simulink model "double_pendulum"  (R2021b)
settings: Solver=VariableStepAuto  StartTime=0.0  StopTime=10.0  RelTol=1e-3
values from neighbouring files (symbols this model uses):
  b1 = 7.7210    (= 7.721)    [benchmark_dbl_pend.m]    (also in dbl_pend_upup_stab_RL.m = 4.8)
  b2 = 2.337424773114795e-05    (= 2.33742477311e-05)    [benchmark_dbl_pend.m]    (also in dbl_pend_upup_stab_RL.m = 0.0002)
  bounds_th1 = [-pi, 3*pi]    [dbl_pend_upup_stab_RL.m]
  c1 = -0.0320    (= -0.032)    [benchmark_dbl_pend.m]    (also in dbl_pend_upup_stab_RL.m = -0.04)
  c2 = 0.053232610186913    (= 0.0532326101869)    [benchmark_dbl_pend.m]    (also in dbl_pend_upup_stab_RL.m = 0.06)
  I1 = 0.0888    [benchmark_dbl_pend.m]    (also in dbl_pend_upup_stab_RL.m = 0.074)
  I2 = 9.5326e-05    [benchmark_dbl_pend.m]    (also in dbl_pend_upup_stab_RL.m = 0.00012)
  km = 53.049364666321930    (= 53.0493646663)    [benchmark_dbl_pend.m]    (also in dbl_pend_upup_stab_RL.m = 50)
  l1 = 0.1    [benchmark_dbl_pend.m]    (also in dbl_pend_upup_stab_RL.m)
  l2 = 0.1    [benchmark_dbl_pend.m]    (also in dbl_pend_upup_stab_RL.m)
  m1 = 0.125    [benchmark_dbl_pend.m]    (also in dbl_pend_upup_stab_RL.m)
  m2 = 0.0493    [benchmark_dbl_pend.m]    (also in dbl_pend_upup_stab_RL.m = 0.05)
  tau_e = 0.014999999999983    (= 0.015)    [benchmark_dbl_pend.m]    (also in dbl_pend_upup_stab_RL.m = 0.03)
  w = [1, 1, 0.05, 0.1]    [dbl_pend_upup_stab_RL.m]
undefined symbols (not defined in the file or in its folder): bounds_th1d, bounds_th2, bounds_th2d, th0, thd0
libraries: simulink x5, rllib x1
settings Model: Creator=MICHAEL-LT  LastModifiedBy=MICHAEL-LT

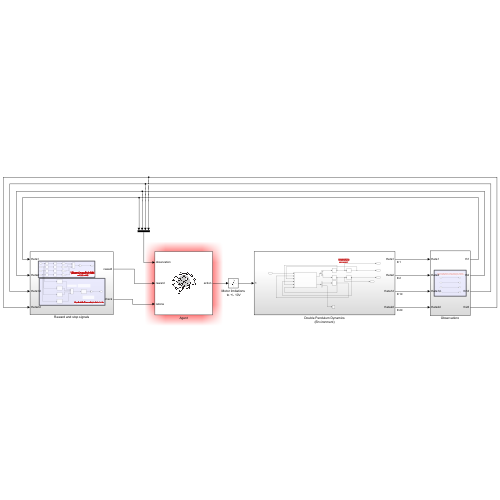
[thumbnail: Simulink's stored preview of the top-level diagram]
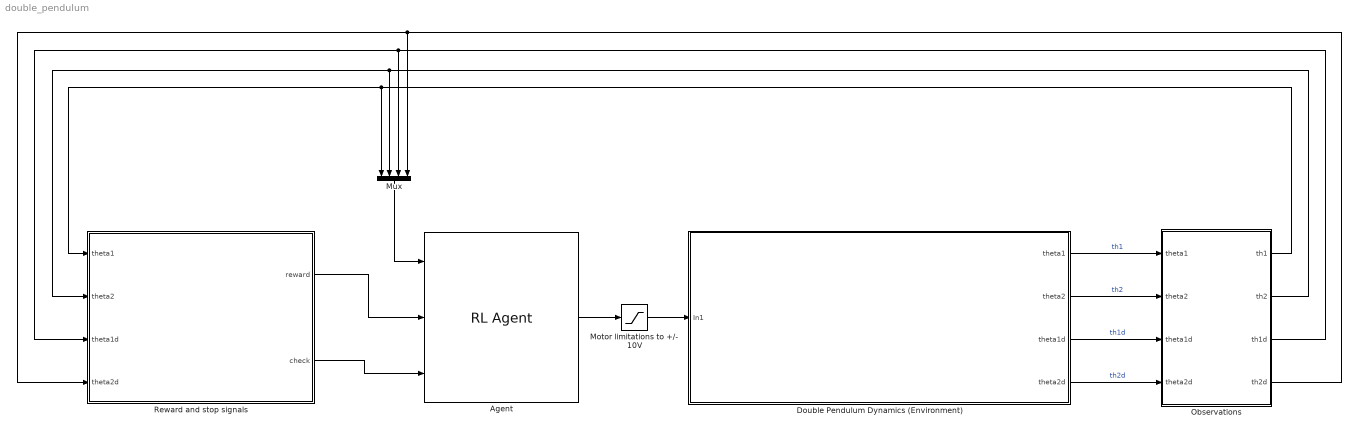
== system double_pendulum ==
  Agent : rllib/RL Agent  Agent=agentObj  ExternalActionAsInput=off  ProvideCumRwd=off  TreatAsDirectFeedthrough=on
  Double Pendulum Dynamics (Environment) : Subsystem
  Motor limitations to +/- 10V : Saturate  UpperLimit=10  LowerLimit=-10
  Mux : Mux
  Observations : Subsystem
  Reward and stop signals : Subsystem
  wires:
  Double Pendulum Dynamics (Environment)/2(theta2) -> Observations/2(theta2)  "th2"
  Double Pendulum Dynamics (Environment)/3(theta1d) -> Observations/3(theta1d)  "th1d"
  Double Pendulum Dynamics (Environment)/1(theta1) -> Observations/1(theta1)  "th1"
  Double Pendulum Dynamics (Environment)/4(theta2d) -> Observations/4(theta2d)  "th2d"
  Observations/2(th2) -> Mux/2, Reward and stop signals/2(theta2)
  Observations/3(th1d) -> Mux/3, Reward and stop signals/3(theta1d)
  Observations/1(th1) -> Mux/1, Reward and stop signals/1(theta1)
  Observations/4(th2d) -> Mux/4, Reward and stop signals/4(theta2d)
  Reward and stop signals/1(reward) -> Agent/2
  Reward and stop signals/2(check) -> Agent/3
  Mux/1 -> Agent/1
  Agent/1 -> Motor limitations to +/- 10V/1
  Motor limitations to +/- 10V/1 -> Double Pendulum Dynamics (Environment)/1(In1)

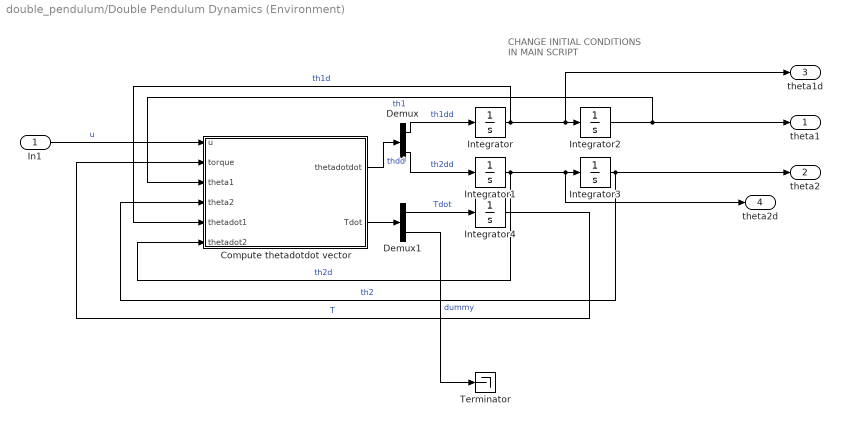
== system double_pendulum/Double Pendulum Dynamics (Environment) ==
  note: CHANGE INITIAL CONDITIONS IN MAIN SCRIPT
  In1 : Inport
  Compute thetadotdot vector : MATLAB Function  TreatAsAtomicUnit=on
  Demux : Demux  Outputs=2
  Demux1 : Demux  Outputs=2
  Integrator : Integrator  InitialCondition=thd0(1)
  Integrator1 : Integrator  InitialCondition=thd0(2)
  Integrator2 : Integrator  InitialCondition=th0(1)
  Integrator3 : Integrator  InitialCondition=th0(2)
  Integrator4 : Integrator
  Terminator : Terminator
  theta1 : Outport
  theta2 : Outport  Port=2
  theta1d : Outport  Port=3
  theta2d : Outport  Port=4
  wires:
  Integrator1/1 -> Compute thetadotdot vector/6(thetadot2), theta2d/1, Integrator3/1  "th2d"
  Integrator4/1 -> Compute thetadotdot vector/2(torque)  "T"
  Demux1/2 -> Terminator/1  "dummy"
  Compute thetadotdot vector/2(Tdot) -> Demux1/1
  In1/1 -> Compute thetadotdot vector/1(u)  "u"
  Compute thetadotdot vector/1(thetadotdot) -> Demux/1  "thdd"
  Integrator/1 -> Compute thetadotdot vector/5(thetadot1), theta1d/1, Integrator2/1  "th1d"
  Integrator3/1 -> theta2/1, Compute thetadotdot vector/4(theta2)  "th2"
  Demux1/1 -> Integrator4/1  "Tdot"
  Integrator2/1 -> Compute thetadotdot vector/3(theta1), theta1/1  "th1"
  Demux/2 -> Integrator1/1  "th2dd"
  Demux/1 -> Integrator/1  "th1dd"

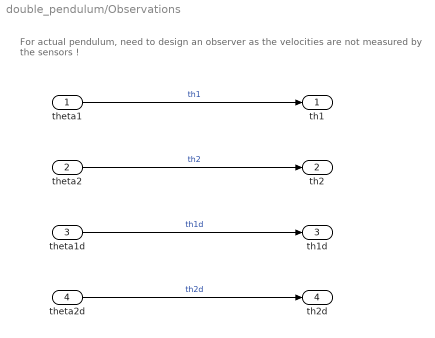
== system double_pendulum/Observations ==
  note: For actual pendulum, need to design an observer
      | as the velocities are not measured by the sensors !
  theta1 : Inport
  theta2 : Inport  Port=2
  theta1d : Inport  Port=3
  theta2d : Inport  Port=4
  th1 : Outport
  th2 : Outport  Port=2
  th1d : Outport  Port=3
  th2d : Outport  Port=4
  wires:
  theta1/1 -> th1/1  "th1"
  theta2/1 -> th2/1  "th2"
  theta1d/1 -> th1d/1  "th1d"
  theta2d/1 -> th2d/1  "th2d"

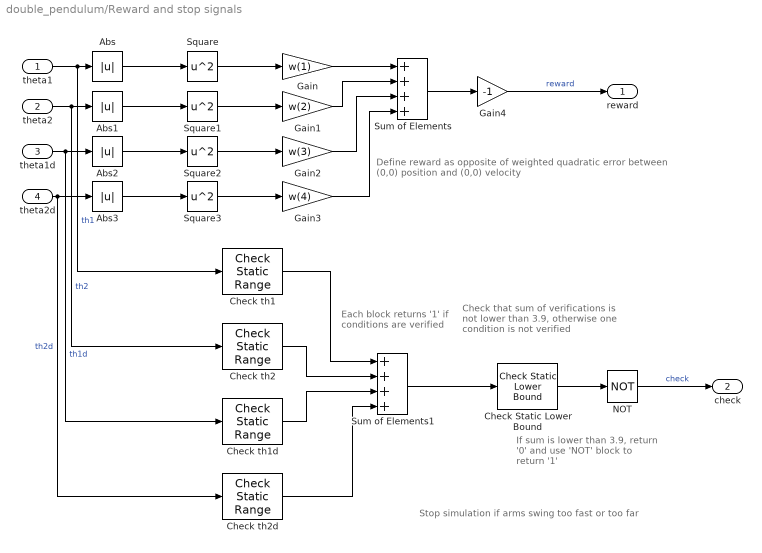
== system double_pendulum/Reward and stop signals ==
  note: Each block returns '1'
      | if conditions are verified
  note: Define reward as opposite of weighted
      | quadratic error between (0,0) position
      | and (0,0) velocity
  note: Stop simulation if arms swing too fast or too far
  note: Check that sum of verifications
      | is not lower than 3.9, otherwise
      | one condition is not verified
  note: If sum is lower than 3.9,
      | return '0' and use 'NOT' block
      | to return '1'
  theta1 : Inport
  theta2 : Inport  Port=2
  theta1d : Inport  Port=3
  theta2d : Inport  Port=4
  Abs{,1..3} (4 alike) : Abs
  Check Static Lower Bound : simulink/Model Verification/Check Static  Lower Bound  Description=3.9 <= u  min=3.9  min_included=on  enabled=on  stopWhenAssertionFail=off  export=on  icon=graphic
  Check th1 : simulink/Model Verification/Check  Static Range  Description=bounds_th1(1) <= u <= bounds_th1(2)  max=bounds_th1(2)  max_included=on  min=bounds_th1(1)  min_included=on  enabled=on  stopWhenAssertionFail=off  export=on  icon=graphic
      settings: SourceProductBaseCode=SL
  Check th1d : simulink/Model Verification/Check  Static Range  Description=bounds_th1d(1) <= u <= bounds_th1d(2)  max=bounds_th1d(2)  max_included=on  min=bounds_th1d(1)  min_included=on  enabled=on  stopWhenAssertionFail=off  export=on  icon=graphic
      settings: SourceProductBaseCode=SL
  Check th2 : simulink/Model Verification/Check  Static Range  Description=bounds_th2(1) <= u <= bounds_th2(2)  max=bounds_th2(2)  max_included=on  min=bounds_th2(1)  min_included=on  enabled=on  stopWhenAssertionFail=off  export=on  icon=graphic
      settings: SourceProductBaseCode=SL
  Check th2d : simulink/Model Verification/Check  Static Range  Description=bounds_th2d(1) <= u <= bounds_th2d(2)  max=bounds_th2d(2)  max_included=on  min=bounds_th2d(1)  min_included=on  enabled=on  stopWhenAssertionFail=off  export=on  icon=graphic
      settings: SourceProductBaseCode=SL
  Gain : Gain  Gain=w(1)
  Gain1 : Gain  Gain=w(2)
  Gain2 : Gain  Gain=w(3)
  Gain3 : Gain  Gain=w(4)
  Gain4 : Gain  Gain=-1
  NOT : Logic  Operator=NOT  IconShape=distinctive  AllPortsSameDT=off  OutDataTypeStr=boolean
  Square{,1..3} (4 alike) : Math  Operator=square  SaturateOnIntegerOverflow=on
  Sum of Elements : Sum  Inputs=++++
  Sum of Elements1 : Sum  Inputs=++++
  reward : Outport
  check : Outport  Port=2
  wires:
  Square/1 -> Gain/1
  Square1/1 -> Gain1/1
  Square2/1 -> Gain2/1
  Square3/1 -> Gain3/1
  theta2d/1 -> Check th2d/1, Abs3/1  "th2d"
  theta1d/1 -> Abs2/1, Check th1d/1  "th1d"
  theta2/1 -> Check th2/1, Abs1/1  "th2"
  theta1/1 -> Check th1/1, Abs/1  "th1"
  Abs/1 -> Square/1
  Abs1/1 -> Square1/1
  Abs2/1 -> Square2/1
  Abs3/1 -> Square3/1
  Gain/1 -> Sum of Elements/1
  Gain1/1 -> Sum of Elements/2
  Gain2/1 -> Sum of Elements/3
  Gain3/1 -> Sum of Elements/4
  Sum of Elements/1 -> Gain4/1
  Gain4/1 -> reward/1  "reward"
  Check th1/1 -> Sum of Elements1/1
  Check th2/1 -> Sum of Elements1/2
  Check th1d/1 -> Sum of Elements1/3
  Check th2d/1 -> Sum of Elements1/4
  Sum of Elements1/1 -> Check Static Lower Bound/1
  Check Static Lower Bound/1 -> NOT/1
  NOT/1 -> check/1  "check"

== matlab function double_pendulum/Double Pendulum Dynamics (Environment)/Compute thetadotdot vector ==
  data: u input; torque input; thetadotdot output; theta1 input; theta2 input; thetadot1 input; thetadot2 input; l1 parameter; l2 parameter; m1 parameter; m2 parameter; c1 parameter; c2 parameter; I1 parameter; I2 parameter; b1 parameter; b2 parameter; km parameter; Tdot output; tau_e parameter
function [thetadotdot, Tdot]  = get_thetadotdot(u, torque, theta1, theta2, thetadot1, thetadot2, l1, l2, m1, m2, c1, c2, I1, I2, b1, b2, km, tau_e)
%% Parameters (SI Units)
g = 9.81;
%% Variables of the model
th1 = theta1;
th2 = theta2;
th1d = thetadot1;
th2d = thetadot2;
thd_vec = [th1d ; th2d];
thetadotdot = [0 ; 0];
T_vec = [torque ; 0];

%% Matrices of physical model
P1 = m1 * c1 * c1 + m2 * l1 * l1 + I1;
P2 = m2 * c2 * c2 + I2;
P3 = m2 * l1 * c2;
g1 = (m1 * c1 + m2 * l1) * g;
g2 = m2 * c2 * g;

M = [[P1 + P2 + 2*P3*cos(th2), P2 + P3 * cos(th2)]; [P2 + P3 * cos(th2) P2]];
C = [[b1 - P3 * th2d * sin(th2), -P3 * (th1d + th2d)*sin(th2)]; [P3 * th1d * sin(th2), b2]];
G = [- g1 * sin(th1) - g2 * sin(th1 + th2); - g2 * sin(th1 + th2)];

%% Compute output angular acceleration
M_inv = inv(M);
Tdot = (km*u - T_vec)/tau_e;
thetadotdot = M_inv*T_vec - M_inv*C*thd_vec - M_inv*G;
